simulink model "SinglePhaseFullWaveRectifierwithTransformer"  (R2020a)
settings: Solver=VariableStepAuto  StartTime=0.0  StopTime=0.0333  RelTol=1e-3
libraries: powerlib x10
settings Model: Creator=Naeem Mohammad  LastModifiedBy=Naeem Mohammad

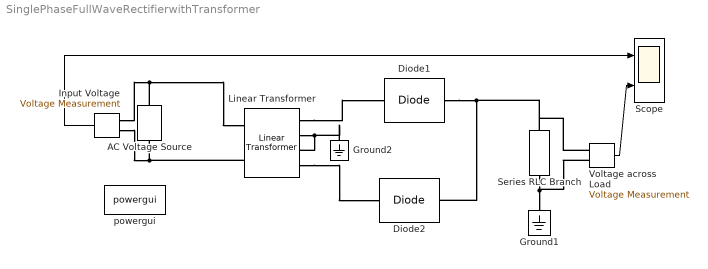
== system SinglePhaseFullWaveRectifierwithTransformer ==
  AC Voltage Source : powerlib/Electrical Sources/AC Voltage Source  Amplitude=110  Phase=0  Frequency=60  SampleTime=0  Measurements=None  BusType=swing  Pref=10e3  Qref=0  Qmin=-inf  Qmax=+inf
  Diode1 : powerlib/Power Electronics/Diode  Ron=0.001  Lon=0  Vf=0.8  IC=0  UseSnubber=0  Rs=500  Cs=250e-9  Measurements=off
  Diode2 : powerlib/Power Electronics/Diode  Ron=0.001  Lon=0  Vf=0.8  IC=0  UseSnubber=0  Rs=500  Cs=250e-9  Measurements=off
  Ground1 : powerlib/Elements/Ground  LConnTagsString=a
  Ground2 : powerlib/Elements/Ground  LConnTagsString=a
  "Input Voltage " : powerlib/Measurements/Voltage Measurement  PhasorSimulation=off  OutputType=Complex  PSBequivalent=0
  Linear Transformer : powerlib/Elements/Linear Transformer  UNITS=pu  NominalPower=[40 60 ]  winding1="[110  0.002  0.08 ]"  winding2="[ 12  0.002  0.08 ]"  ThreeWindings=on  winding3=[ 12 0.002 0.08 ]  RmLm=[ 500 500 ]  Measurements=None  DataType=off
  Scope : Scope  NumInputPorts=2
  Series RLC Branch : powerlib/Elements/Series RLC Branch  LConnTagsString=__new0  RConnTagsString=__new0  BranchType=R  Resistance=10  Inductance=1e-3  SetiL0=off  InitialCurrent=0  Capacitance=1e-6  Setx0=off  InitialVoltage=0  Measurements=None
  Voltage across Load : powerlib/Measurements/Voltage Measurement  PhasorSimulation=off  OutputType=Complex  PSBequivalent=0
  powergui : powerlib/powergui  Priority=1  SimulationMode=Continuous  SampleTime=50e-6  frequency=60  Iterations=50  frequencyindice=60  Pbase=100e6  ErrMax=1e-4  UnitsV=kV  UnitsW=MW  buscounter=0  FunctionMessages=off  echomessages=off  EnableUseOfTLC=off  CurrentSourceSwitches=off  DisableSnubberDevices=off  DisableRonSwitches=off  DisableVfSwitches=off  DisplayEquations=off  AutomaticDiscreteSolvers=off  SolverType=Tustin/Backward Euler (TBE)  Interpol=off  ExternalGateDelay=off  methode=off  Ts=100  x0status=blocks  SPID=on  SwTol=0  HookPort=off  NonlinearTolerance=1e-4  nMaxIteration=100  ContinueOnMaxIteration=off  RestoreLinks=warning  ResistiveCurrentMeasurement=off  Frange=[0:2:500]  Ylog=off  Xlog=on  ShowGrid=off  save=off  variable=ZData  structure=0  ZoomFFT=off  StartTime=0.0  cycles=1  DisplayStyle=1  fundamental=60  FreqAxis=off  MaxFrequency=1000  frequencyindicesteady=1  RmsSteady=1  display=off
  wires:
  Voltage across Load/1 -> Scope/2
  "Input Voltage "/1 -> Scope/1
  connections:
  Diode1/RConn1 -- Voltage across Load/LConn1 -- Series RLC Branch/LConn1 -- Diode2/RConn1
  "Input Voltage "/LConn2 -- Linear Transformer/LConn2 -- AC Voltage Source/LConn1
  "Input Voltage "/LConn1 -- AC Voltage Source/RConn1 -- Linear Transformer/LConn1
  Linear Transformer/RConn1 -- Diode1/LConn1
  Series RLC Branch/RConn1 -- Voltage across Load/LConn2 -- Ground1/LConn1
  Linear Transformer/RConn4 -- Diode2/LConn1
  Linear Transformer/RConn2 -- Linear Transformer/RConn3 -- Ground2/LConn1
